simulink model "three_tank_ideal_ver1_2013"  (R2013a)
settings: Solver=ode45  StartTime=0.0  StopTime=15000  RelTol=1e-3
settings Model: Creator=safaeipour  LastModifiedBy=hossein
settings SolverCC: ZeroCrossAlgorithm=Adaptive
settings DataIOCC: SaveFormat=StructureWithTime
settings DebuggingCC: UnderspecifiedInitializationDetection=Simplified  MergeDetectMultiDrivingBlocksExec=error  IgnoredZcDiagnostic=none  SolverPrmCheckMsg=none  FrameProcessingCompatibilityMsg=error  StateNameClashWarn=none
settings HardwareCC: ProdBitPerPointer=64  ProdLargestAtomicFloat=Float  ProdIntDivRoundTo=Zero  ProdEndianess=LittleEndian  ProdHWDeviceType=Specified
settings GRTTargetCC: CodeReplacementLibrary=C89/C90 (ANSI)  GeneratePreprocessorConditionals=Use local settings
settings ConfigurationSet: Description=Simscape Multibody

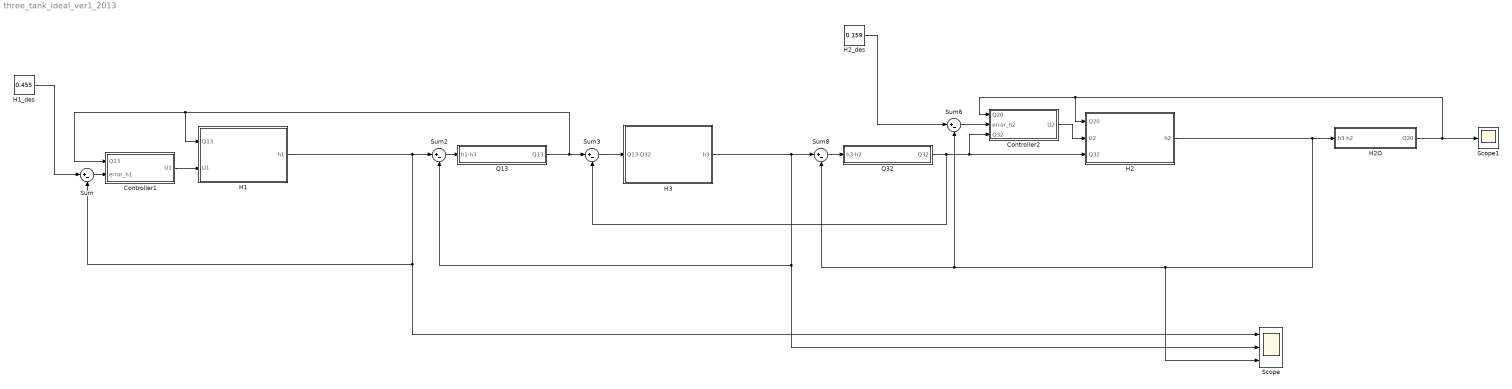
== system three_tank_ideal_ver1_2013 ==
  Controller1 : Subsystem
  Controller2 : Subsystem
  H1 : Subsystem
  "H1_des " : Constant  Value=0.455
  H2 : Subsystem
  H2O : Subsystem
  H2_des : Constant  Value=0.159
  H3 : Subsystem
  Q13 : Subsystem
  Q32 : Subsystem
  Scope : Scope  NumInputPorts=3
      settings: TimeRange=auto  MaxDataPoints=5000  SaveToWorkspace=off  YMin=0.44838~-0.04011~-0.01997  YMax=0.46127~0.36098~0.17977  SampleTime=-1
  Scope1 : Scope
      settings: TimeRange=auto  MaxDataPoints=5000  SaveToWorkspace=off  SaveName=ScopeData2  YMin=-0.000005  YMax=0.000061  SampleTime=-1
  Sum{,2..3,6,8} (5 alike) : Sum  Inputs=|+-
  wires:
  Q13/1(Q13) -> H1/1(Q13), Controller1/1(Q13), Sum3/1
  Sum6/1 -> Controller2/2(error_h2)
  Q32/1(Q32) -> Controller2/3(Q32), H2/3(Q32), Sum3/2
  Sum3/1 -> H3/1(Q13-Q32)
  "H1_des "/1 -> Sum/1
  H2_des/1 -> Sum6/1
  Sum2/1 -> Q13/1(h1-h3)
  Sum8/1 -> Q32/1(h3-h2)
  Sum/1 -> Controller1/2(error_h1)
  H2O/1(Q20) -> Controller2/1(Q20), H2/1(Q20), Scope1/1
  H1/1(h1) -> Scope/1, Sum/2, Sum2/1
  H3/1(h3) -> Scope/2, Sum2/2, Sum8/1
  H2/1(h2) -> Scope/3, Sum8/2, Sum6/2, H2O/1(h3-h2)
  Controller1/1(U1) -> H1/2(U1)
  Controller2/1(U2) -> H2/2(U2)

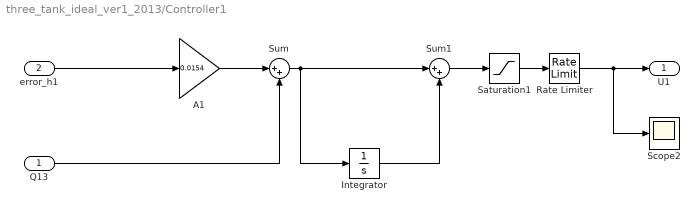
== system three_tank_ideal_ver1_2013/Controller1 ==
  Q13 : Inport
  error_h1 : Inport  Port=2
  A1 : Gain  Gain=0.0154
  Integrator : Integrator  ZeroCross=off
  Rate Limiter : RateLimiter  RisingSlewLimit=0.000000008  FallingSlewLimit=-0.000000008  SampleTimeMode=inherited  LinearizeAsGain=off
  Saturation1 : Saturate  UpperLimit=0.00004  LowerLimit=0.00000  ZeroCross=off
  Scope2 : Scope
      settings: TimeRange=auto  MaxDataPoints=5000  SaveToWorkspace=off  YMin=-0.000005  YMax=0.000045  SampleTime=-1
  Sum : Sum  Inputs=|++
  Sum1 : Sum  Inputs=|++
  U1 : Outport
  wires:
  error_h1/1 -> A1/1
  Rate Limiter/1 -> U1/1, Scope2/1
  A1/1 -> Sum/1
  Q13/1 -> Sum/2
  Sum1/1 -> Saturation1/1
  Integrator/1 -> Sum1/2
  Saturation1/1 -> Rate Limiter/1
  Sum/1 -> Integrator/1, Sum1/1

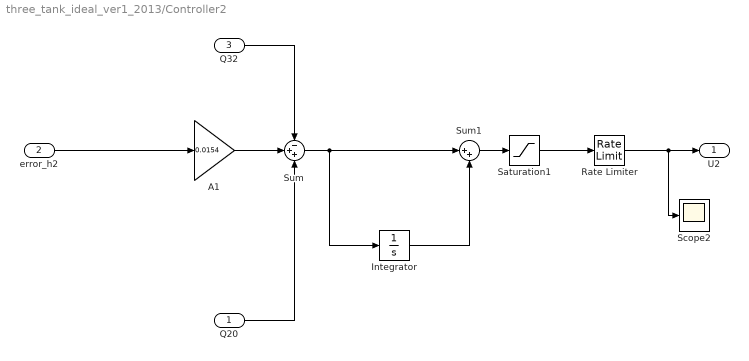
== system three_tank_ideal_ver1_2013/Controller2 ==
  Q20 : Inport
  error_h2 : Inport  Port=2
  Q32 : Inport  Port=3
  A1 : Gain  Gain=0.0154
  Integrator : Integrator  ZeroCross=off
  Rate Limiter : RateLimiter  RisingSlewLimit=0.000000008  FallingSlewLimit=-0.000000008  SampleTimeMode=inherited  LinearizeAsGain=off
  Saturation1 : Saturate  UpperLimit=0.000014  LowerLimit=0.00000  ZeroCross=off
  Scope2 : Scope
      settings: TimeRange=auto  MaxDataPoints=5000  SaveToWorkspace=off  YMin=0.000013925  YMax=0.000014008  SampleTime=-1
  Sum : Sum  Inputs=-++
  Sum1 : Sum  Inputs=|++
  U2 : Outport
  wires:
  Rate Limiter/1 -> U2/1, Scope2/1
  error_h2/1 -> A1/1
  Saturation1/1 -> Rate Limiter/1
  A1/1 -> Sum/2
  Q32/1 -> Sum/1
  Q20/1 -> Sum/3
  Integrator/1 -> Sum1/2
  Sum/1 -> Integrator/1, Sum1/1
  Sum1/1 -> Saturation1/1

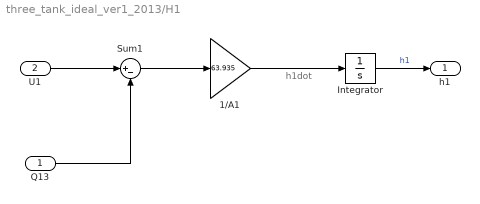
== system three_tank_ideal_ver1_2013/H1 ==
  note: h1dot
  Q13 : Inport
  U1 : Inport  Port=2
  1/A1 : Gain  Gain=63.935
  Integrator : Integrator  ZeroCross=off
  Sum1 : Sum  Inputs=|+-
  h1 : Outport
  wires:
  Sum1/1 -> 1/A1/1
  Q13/1 -> Sum1/2
  Integrator/1 -> h1/1  "h1"
  U1/1 -> Sum1/1
  1/A1/1 -> Integrator/1

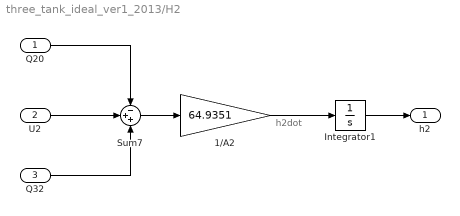
== system three_tank_ideal_ver1_2013/H2 ==
  note: h2dot
  Q20 : Inport
  U2 : Inport  Port=2
  Q32 : Inport  Port=3
  1/A2 : Gain  Gain=64.9351
  Integrator1 : Integrator
  Sum7 : Sum  Inputs=-++
  h2 : Outport
  wires:
  Sum7/1 -> 1/A2/1
  Integrator1/1 -> h2/1
  Q32/1 -> Sum7/3
  Q20/1 -> Sum7/1
  U2/1 -> Sum7/2
  1/A2/1 -> Integrator1/1

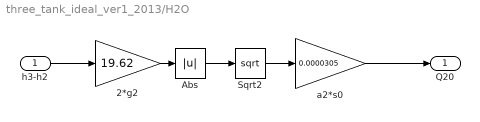
== system three_tank_ideal_ver1_2013/H2O ==
  h3-h2 : Inport
  2*g2 : Gain  Gain=19.62
  Abs : Abs  ZeroCross=off
  Sqrt2 : Sqrt  SaturateOnIntegerOverflow=on
  a2*s0 : Gain  Gain=0.0000305
  Q20 : Outport
  wires:
  2*g2/1 -> Abs/1
  Sqrt2/1 -> a2*s0/1
  a2*s0/1 -> Q20/1
  h3-h2/1 -> 2*g2/1
  Abs/1 -> Sqrt2/1

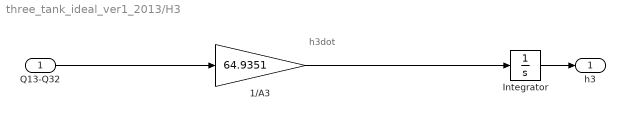
== system three_tank_ideal_ver1_2013/H3 ==
  note: h3dot
  Q13-Q32 : Inport
  1/A3 : Gain  Gain=64.9351
  Integrator : Integrator  ZeroCross=off
  h3 : Outport
  wires:
  1/A3/1 -> Integrator/1
  Integrator/1 -> h3/1
  Q13-Q32/1 -> 1/A3/1

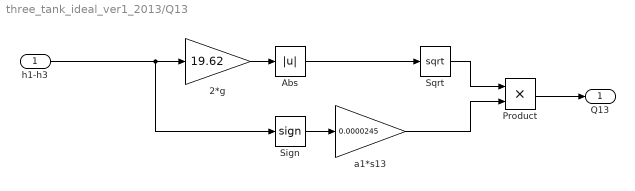
== system three_tank_ideal_ver1_2013/Q13 ==
  h1-h3 : Inport
  2*g : Gain  Gain=19.62
  Abs : Abs  ZeroCross=off
  Product : Product
  Sign : Signum  ZeroCross=off
  Sqrt : Sqrt  SaturateOnIntegerOverflow=on
  "a1*s13 " : Gain  Gain=0.0000245
  Q13 : Outport
  wires:
  "a1*s13 "/1 -> Product/2
  h1-h3/1 -> Sign/1, 2*g/1
  Abs/1 -> Sqrt/1
  Sqrt/1 -> Product/1
  Sign/1 -> "a1*s13 "/1
  Product/1 -> Q13/1
  2*g/1 -> Abs/1

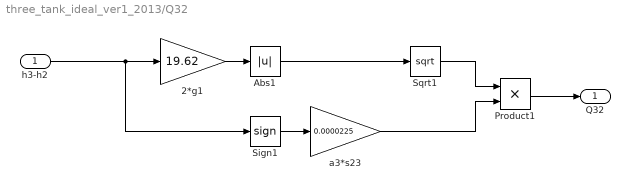
== system three_tank_ideal_ver1_2013/Q32 ==
  h3-h2 : Inport
  2*g1 : Gain  Gain=19.62
  Abs1 : Abs  ZeroCross=off
  Product1 : Product
  Sign1 : Signum  ZeroCross=off
  Sqrt1 : Sqrt  SaturateOnIntegerOverflow=on
  a3*s23 : Gain  Gain=0.0000225
  Q32 : Outport
  wires:
  h3-h2/1 -> Sign1/1, 2*g1/1
  Sign1/1 -> a3*s23/1
  Abs1/1 -> Sqrt1/1
  Sqrt1/1 -> Product1/1
  a3*s23/1 -> Product1/2
  Product1/1 -> Q32/1
  2*g1/1 -> Abs1/1
